simulink model "OneZeroOneDetector"  (R2025b)
settings: Solver=FixedStepDiscrete  StartTime=0.0  StopTime=Inf  RelTol=1e-3
settings Model: Creator=Soochan Kim  LastModifiedBy=Soochan Kim
settings OptimizationCC: BlockReduction=off  ConditionallyExecuteInputs=off  DefaultParameterBehavior=Inlined
settings DebuggingCC: AlgebraicLoopMsg=error
settings HardwareCC: ProdBitPerPointer=32.0  ProdBitPerSizeT=32.0  ProdBitPerPtrDiffT=32.0  ProdLargestAtomicFloat=None  ProdIntDivRoundTo=Undefined  ProdEndianess=Unspecified  ProdWordSize=32.0  ProdHWDeviceType=ASIC/FPGA->ASIC/FPGA  TargetBitPerPointer=64.0  TargetBitPerSizeT=64.0  TargetBitPerPtrDiffT=64.0  TargetLongLongMode=on  TargetIntDivRoundTo=Zero  TargetEndianess=LittleEndian  TargetWordSize=64.0  TargetHWDeviceType=Custom Processor->MATLAB Host Computer  ProdEqTarget=off

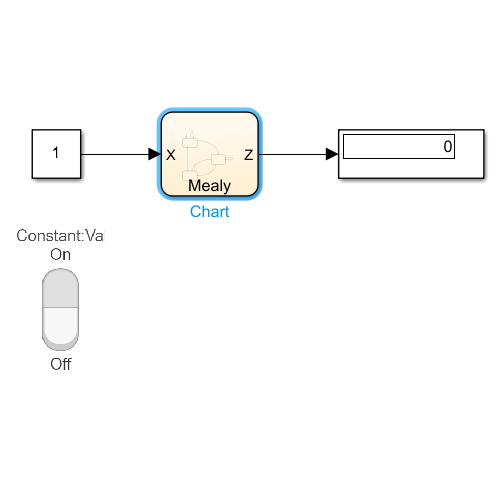
[thumbnail: Simulink's stored preview of the top-level diagram]
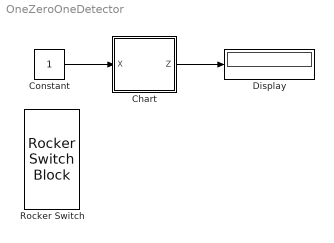
== system OneZeroOneDetector ==
  Chart : Stateflow chart  TreatAsAtomicUnit=on
  Constant : Constant  OutDataTypeStr=boolean
  Display : Display
  Rocker Switch : RockerSwitchBlock
  wires:
  Chart/1(Z) -> Display/1
  Constant/1 -> Chart/1(X)

== stateflow chart OneZeroOneDetector/Chart ==
  settings: updateMethod=DISCRETE  sampleTime=1  stateMachineType=MEALY_MACHINE  executeAtInitialization=1  initializeOutput=1
  state S0
  state S1
  state S2
  S0 -> S0 [order 2] : [X==false]{Z=false}
  (default) -> S0
  S0 -> S1 [order 1] : [X==true]{Z=false}
  S2 -> S0 [order 2] : [X==false]{Z=false}
  S1 -> S1 [order 1] : [X==true]{Z=false}
  S2 -> S1 [order 1] : [X==true]{Z=true}
  S1 -> S2 [order 2] : [X==false]{Z=false}
  data: X input boolean; Z output boolean
